simulink model "TRMS_Model"  (R2023b)
settings: Solver=FixedStepAuto  StartTime=0.0  StopTime=70  FixedStep=1e-5  RelTol=1e-3
libraries: slpidlib x2
settings Model: Creator=user  LastModifiedBy=user

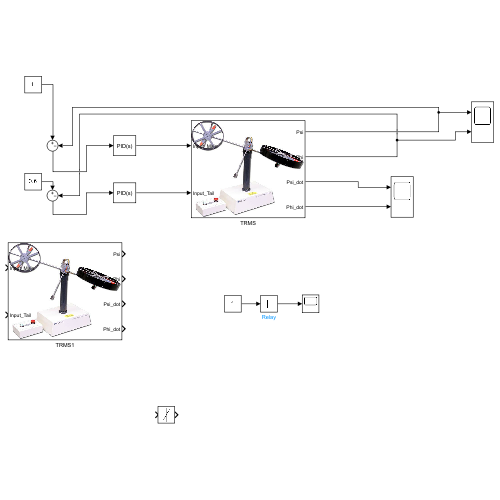
[thumbnail: Simulink's stored preview of the top-level diagram]
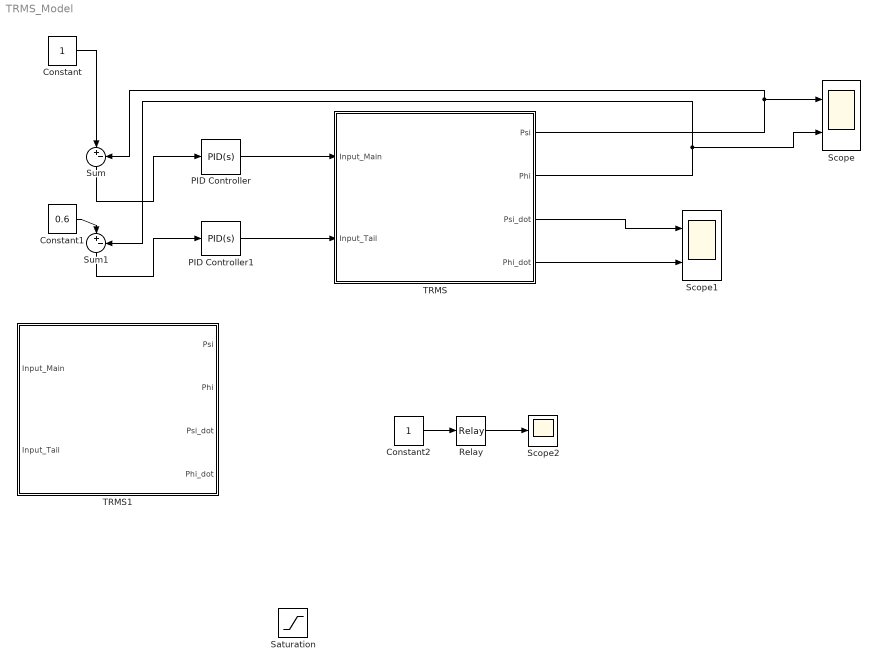
== system TRMS_Model ==
  Constant : Constant
  Constant1 : Constant  Value=0.6
  Constant2 : Constant
  PID Controller : slpidlib/PID Controller  Controller=PID  Form=Parallel  TimeDomain=Continuous-time  UseExternalTs=off  SampleTime=-1  IntegratorMethod=Forward Euler  FilterMethod=Forward Euler  ControllerParametersSource=internal  P=0  I=0.40844029645165  UseKiTs=off  D=0  N=100  UseFilter=on  TunerSelectOption=Transfer Function Based (PID Tuner App)  InitialConditionSource=internal  InitialConditionForIntegrator=0  InitialConditionForFilter=0  DifferentiatorICPrevScaledInput=0  ExternalReset=none  TrackingMode=off  Kt=1  LimitOutput=off  SatLimitsSource=internal  UpperSaturationLimit=inf  LowerSaturationLimit=-inf  LinearizeAsGain=on  AntiWindupMode=none  Kb=1  LimitIntegrator=off  UpperIntegratorSaturationLimit=inf  LowerIntegratorSaturationLimit=-inf  POutMin=[]  POutMax=[]  IOutMin=[]  IOutMax=[]  DOutMin=[]  DOutMax=[]  NOutMin=[]  NOutMax=[]  SumOutMin=[]  SumOutMax=[]  SaturationOutMin=[]  SaturationOutMax=[]  PParamMin=[]  PParamMax=[]  IParamMin=[]  IParamMax=[]  DParamMin=[]  DParamMax=[]  NParamMin=[]  NParamMax=[]  KbParamMin=[]  KbParamMax=[]  KtParamMin=[]  KtParamMax=[]  KbOutMin=[]  KbOutMax=[]  KtOutMin=[]  KtOutMax=[]  IntegratorOutMin=[]  IntegratorOutMax=[]  FilterOutMin=[]  FilterOutMax=[]  SumI1OutMin=[]  SumI1OutMax=[]  SumI2OutMin=[]  SumI2OutMax=[]  SumI3OutMin=[]  SumI3OutMax=[]  SumI4OutMin=[]  SumI4OutMax=[]  SumDOutMin=[]  SumDOutMax=[]  DifferentiatorOutMin=[]  DifferentiatorOutMax=[]  FilterDiffOutCoefMin=[]  FilterDiffOutCoefMax=[]  ReciprocalOutMin=[]  ReciprocalOutMax=[]  SumDenOutMin=[]  SumDenOutMax=[]  SumNumOutMin=[]  SumNumOutMax=[]  DivideOutMin=[]  DivideOutMax=[]  UdiffTsProdOutMin=[]  UdiffTsProdOutMax=[]  NTsProdOutMin=[]  NTsProdOutMax=[]  UintegralTsProdOutMin=[]  UintegralTsProdOutMax=[]  UngainTsProdOutMin=[]  UngainTsProdOutMax=[]  ClampingZeroOutDataTypeStr=Inherit: Inherit via back propagation  ClampingZeroOutMin=[]  ClampingZeroOutMax=[]  FilterDenConstantOutDataTypeStr=Inherit: Inherit via back propagation  FilterDenConstantOutMin=[]  FilterDenConstantOutMax=[]  PCopyOutDataTypeStr=Inherit: Inherit via back propagation  PCopyOutMin=[]  PCopyOutMax=[]  NCopyOutDataTypeStr=Inherit: Inherit via back propagation  NCopyOutMin=[]  NCopyOutMax=[]  IntegratorContinuousStateAttributes=''  IntegratorStateMustResolveToSignalObject=off  IntegratorRTWStateStorageClass=Auto  FilterContinuousStateAttributes=''  FilterStateMustResolveToSignalObject=off  FilterRTWStateStorageClass=Auto  ParallelPVariant=InternalParameters  IdealPVariant=Disabled  IVariant=InternalParameters  DVariant=InternalParameters  IntegratorVariant=Continuous  SatVariant=Disabled  AWVariant=Passthrough  PCopyVariant=Disabled  TRVariant=Disabled  FdbkBlocksVariant=Forward  IdealPFdbkVariant=Disabled  SatFdbkVariant=Disabled  DerivativeFilterVariant=ContFilter  NVariant=InternalParameters  NCopyVariant=Disabled  FilterICVariant=InternalICsFilter  IntegratorICVariant=InternalICs  ExternalResetVariant=Disabled  TRSumVariant=Passthrough  SumFdbkVariant=Disabled  SumVariant=Sum_PID  TsampFilterVariant=InternalTs  TsampNgainVariant=Passthrough  TsampIntegralVariant=Disabled_SignalSpec  ExternalSaturationOutDataTypeStr=Inherit: Same as second input
  PID Controller1 : slpidlib/PID Controller  Controller=PID  Form=Parallel  TimeDomain=Continuous-time  UseExternalTs=off  SampleTime=-1  IntegratorMethod=Forward Euler  FilterMethod=Forward Euler  ControllerParametersSource=internal  P=4.51040061904311  I=0.763929883616639  UseKiTs=off  D=4.55570625912268  N=321.160537839472  UseFilter=on  TunerSelectOption=Transfer Function Based (PID Tuner App)  InitialConditionSource=internal  InitialConditionForIntegrator=0  InitialConditionForFilter=0  DifferentiatorICPrevScaledInput=0  ExternalReset=none  TrackingMode=off  Kt=1  LimitOutput=off  SatLimitsSource=internal  UpperSaturationLimit=inf  LowerSaturationLimit=-inf  LinearizeAsGain=on  AntiWindupMode=none  Kb=1  LimitIntegrator=off  UpperIntegratorSaturationLimit=inf  LowerIntegratorSaturationLimit=-inf  POutMin=[]  POutMax=[]  IOutMin=[]  IOutMax=[]  DOutMin=[]  DOutMax=[]  NOutMin=[]  NOutMax=[]  SumOutMin=[]  SumOutMax=[]  SaturationOutMin=[]  SaturationOutMax=[]  PParamMin=[]  PParamMax=[]  IParamMin=[]  IParamMax=[]  DParamMin=[]  DParamMax=[]  NParamMin=[]  NParamMax=[]  KbParamMin=[]  KbParamMax=[]  KtParamMin=[]  KtParamMax=[]  KbOutMin=[]  KbOutMax=[]  KtOutMin=[]  KtOutMax=[]  IntegratorOutMin=[]  IntegratorOutMax=[]  FilterOutMin=[]  FilterOutMax=[]  SumI1OutMin=[]  SumI1OutMax=[]  SumI2OutMin=[]  SumI2OutMax=[]  SumI3OutMin=[]  SumI3OutMax=[]  SumI4OutMin=[]  SumI4OutMax=[]  SumDOutMin=[]  SumDOutMax=[]  DifferentiatorOutMin=[]  DifferentiatorOutMax=[]  FilterDiffOutCoefMin=[]  FilterDiffOutCoefMax=[]  ReciprocalOutMin=[]  ReciprocalOutMax=[]  SumDenOutMin=[]  SumDenOutMax=[]  SumNumOutMin=[]  SumNumOutMax=[]  DivideOutMin=[]  DivideOutMax=[]  UdiffTsProdOutMin=[]  UdiffTsProdOutMax=[]  NTsProdOutMin=[]  NTsProdOutMax=[]  UintegralTsProdOutMin=[]  UintegralTsProdOutMax=[]  UngainTsProdOutMin=[]  UngainTsProdOutMax=[]  ClampingZeroOutDataTypeStr=Inherit: Inherit via back propagation  ClampingZeroOutMin=[]  ClampingZeroOutMax=[]  FilterDenConstantOutDataTypeStr=Inherit: Inherit via back propagation  FilterDenConstantOutMin=[]  FilterDenConstantOutMax=[]  PCopyOutDataTypeStr=Inherit: Inherit via back propagation  PCopyOutMin=[]  PCopyOutMax=[]  NCopyOutDataTypeStr=Inherit: Inherit via back propagation  NCopyOutMin=[]  NCopyOutMax=[]  IntegratorContinuousStateAttributes=''  IntegratorStateMustResolveToSignalObject=off  IntegratorRTWStateStorageClass=Auto  FilterContinuousStateAttributes=''  FilterStateMustResolveToSignalObject=off  FilterRTWStateStorageClass=Auto  ParallelPVariant=InternalParameters  IdealPVariant=Disabled  IVariant=InternalParameters  DVariant=InternalParameters  IntegratorVariant=Continuous  SatVariant=Disabled  AWVariant=Passthrough  PCopyVariant=Disabled  TRVariant=Disabled  FdbkBlocksVariant=Forward  IdealPFdbkVariant=Disabled  SatFdbkVariant=Disabled  DerivativeFilterVariant=ContFilter  NVariant=InternalParameters  NCopyVariant=Disabled  FilterICVariant=InternalICsFilter  IntegratorICVariant=InternalICs  ExternalResetVariant=Disabled  TRSumVariant=Passthrough  SumFdbkVariant=Disabled  SumVariant=Sum_PID  TsampFilterVariant=InternalTs  TsampNgainVariant=Passthrough  TsampIntegralVariant=Disabled_SignalSpec  ExternalSaturationOutDataTypeStr=Inherit: Same as second input
  Relay : Relay  OnSwitchValue=0.01  OffSwitchValue=-0.01  OffOutputValue=-1
  Saturation : Saturate
  Scope : Scope  NumInputPorts=2
  Scope1 : Scope  NumInputPorts=2
  Scope2 : Scope
  Sum : Sum  Inputs=|+-
  Sum1 : Sum  Inputs=|+-
  TRMS : Subsystem
      mask Display: image('Twin-Rotor-MIMO-System.png');
  TRMS1 : Subsystem
      mask Display: image('Twin-Rotor-MIMO-System.png');
  wires:
  PID Controller/1 -> TRMS/1(Input_Main)
  Sum/1 -> PID Controller/1
  Constant/1 -> Sum/1
  TRMS/1(Psi) -> Scope/1, Sum/2
  PID Controller1/1 -> TRMS/2(Input_Tail)
  Constant1/1 -> Sum1/1
  Sum1/1 -> PID Controller1/1
  TRMS/2(Phi) -> Scope/2, Sum1/2
  TRMS/3(Psi_dot) -> Scope1/1
  TRMS/4(Phi_dot) -> Scope1/2
  Relay/1 -> Scope2/1
  Constant2/1 -> Relay/1

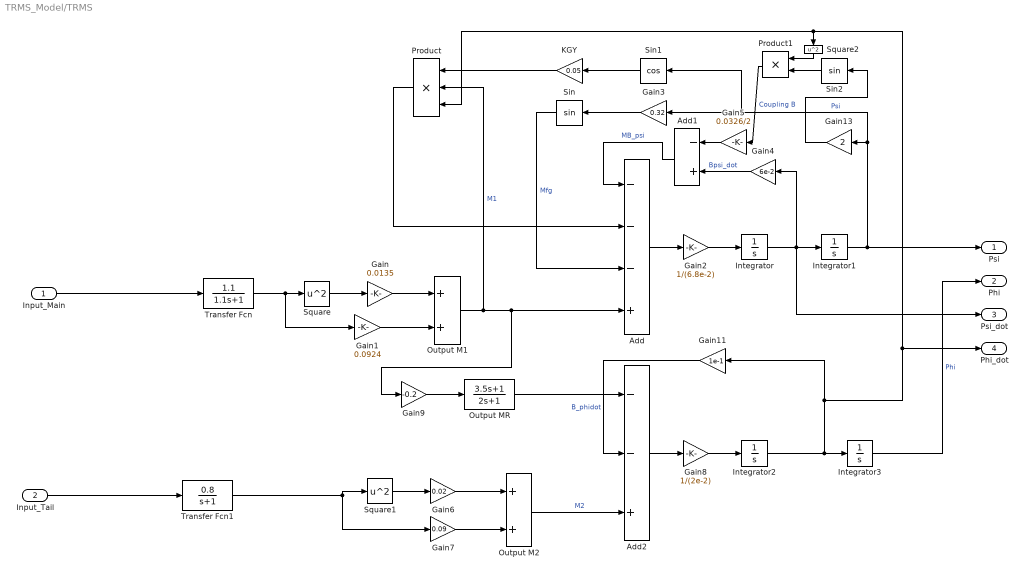
== system TRMS_Model/TRMS ==
  Input_Main : Inport
  Input_Tail : Inport  Port=2
  Add : Sum  Inputs=---+
  Add1 : Sum  Inputs=-+
  Add2 : Sum  Inputs=--+
  Gain : Gain  Gain=0.0135
  Gain1 : Gain  Gain=0.0924
  Gain11 : Gain  Gain=1e-1
  Gain13 : Gain  Gain=2
  Gain2 : Gain  Gain=1/(6.8e-2)
  Gain3 : Gain  Gain=0.32
  Gain4 : Gain  Gain=6e-2
  Gain5 : Gain  Gain=0.0326/2
  Gain6 : Gain  Gain=0.02
  Gain7 : Gain  Gain=0.09
  Gain8 : Gain  Gain=1/(2e-2)
  Gain9 : Gain  Gain=-0.2
  Integrator{,1..3} (4 alike) : Integrator
  KGY : Gain  Gain=0.05
  Output M1 : Sum
  Output M2 : Sum
  Output MR : TransferFcn  Numerator=[3.5 1]  Denominator=[2 1]
  Product : Product  Inputs=3
  Product1 : Product
  Sin : Trigonometry
  Sin1 : Trigonometry  Operator=cos
  Sin2 : Trigonometry
  Square : Math  Operator=square
  Square1 : Math  Operator=square
  Square2 : Math  Operator=square
  Transfer Fcn : TransferFcn  Numerator=[1.1]  Denominator=[1.1 1]
  Transfer Fcn1 : TransferFcn  Numerator=[0.8]  Denominator=[1 1]
  Psi : Outport
  Phi : Outport  Port=2
  Psi_dot : Outport  Port=3
  Phi_dot : Outport  Port=4
  wires:
  Integrator2/1 -> Phi_dot/1, Product/3, Square2/1, Gain11/1, Integrator3/1
  Product1/1 -> Gain5/1  "Coupling B"
  Add1/1 -> Add/1  "MB_psi"
  Integrator1/1 -> Psi/1, Gain13/1, Sin1/1, Gain3/1  "Psi"
  Sin2/1 -> Product1/2
  Product/1 -> Add/2
  Transfer Fcn/1 -> Square/1, Gain1/1
  Square1/1 -> Gain6/1
  Gain3/1 -> Sin/1
  Add/1 -> Gain2/1
  Gain1/1 -> Output M1/2
  Square/1 -> Gain/1
  Gain13/1 -> Sin2/1
  Transfer Fcn1/1 -> Gain7/1, Square1/1
  Integrator/1 -> Psi_dot/1, Gain4/1, Integrator1/1
  Gain/1 -> Output M1/1
  Gain9/1 -> Output MR/1
  Gain6/1 -> Output M2/1
  Output M2/1 -> Add2/3  "M2"
  Output M1/1 -> Gain9/1, Add/4, Product/2  "M1"
  Add2/1 -> Gain8/1
  Sin1/1 -> KGY/1
  Gain2/1 -> Integrator/1
  KGY/1 -> Product/1
  Gain11/1 -> Add2/2  "B_phidot"
  Gain7/1 -> Output M2/2
  Output MR/1 -> Add2/1
  Gain8/1 -> Integrator2/1
  Gain4/1 -> Add1/2  "Bpsi_dot"
  Gain5/1 -> Add1/1
  Input_Main/1 -> Transfer Fcn/1
  Sin/1 -> Add/3  "Mfg"
  Square2/1 -> Product1/1
  Input_Tail/1 -> Transfer Fcn1/1
  Integrator3/1 -> Phi/1  "Phi"

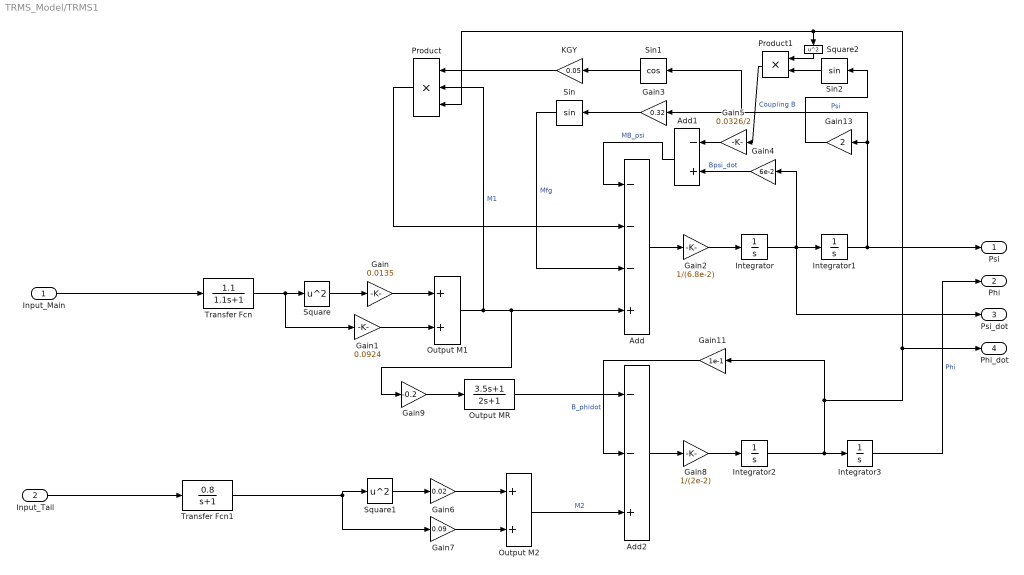
== system TRMS_Model/TRMS1 ==
  Input_Main : Inport
  Input_Tail : Inport  Port=2
  Add : Sum  Inputs=---+
  Add1 : Sum  Inputs=-+
  Add2 : Sum  Inputs=--+
  Gain : Gain  Gain=0.0135
  Gain1 : Gain  Gain=0.0924
  Gain11 : Gain  Gain=1e-1
  Gain13 : Gain  Gain=2
  Gain2 : Gain  Gain=1/(6.8e-2)
  Gain3 : Gain  Gain=0.32
  Gain4 : Gain  Gain=6e-2
  Gain5 : Gain  Gain=0.0326/2
  Gain6 : Gain  Gain=0.02
  Gain7 : Gain  Gain=0.09
  Gain8 : Gain  Gain=1/(2e-2)
  Gain9 : Gain  Gain=-0.2
  Integrator{,1..3} (4 alike) : Integrator
  KGY : Gain  Gain=0.05
  Output M1 : Sum
  Output M2 : Sum
  Output MR : TransferFcn  Numerator=[3.5 1]  Denominator=[2 1]
  Product : Product  Inputs=3
  Product1 : Product
  Sin : Trigonometry
  Sin1 : Trigonometry  Operator=cos
  Sin2 : Trigonometry
  Square : Math  Operator=square
  Square1 : Math  Operator=square
  Square2 : Math  Operator=square
  Transfer Fcn : TransferFcn  Numerator=[1.1]  Denominator=[1.1 1]
  Transfer Fcn1 : TransferFcn  Numerator=[0.8]  Denominator=[1 1]
  Psi : Outport
  Phi : Outport  Port=2
  Psi_dot : Outport  Port=3
  Phi_dot : Outport  Port=4
  wires:
  Integrator3/1 -> Phi/1  "Phi"
  Input_Tail/1 -> Transfer Fcn1/1
  Square2/1 -> Product1/1
  Sin/1 -> Add/3  "Mfg"
  Input_Main/1 -> Transfer Fcn/1
  Gain5/1 -> Add1/1
  Gain4/1 -> Add1/2  "Bpsi_dot"
  Gain8/1 -> Integrator2/1
  Output MR/1 -> Add2/1
  Gain7/1 -> Output M2/2
  Gain11/1 -> Add2/2  "B_phidot"
  KGY/1 -> Product/1
  Gain2/1 -> Integrator/1
  Sin1/1 -> KGY/1
  Add2/1 -> Gain8/1
  Output M1/1 -> Product/2, Add/4, Gain9/1  "M1"
  Output M2/1 -> Add2/3  "M2"
  Gain6/1 -> Output M2/1
  Gain9/1 -> Output MR/1
  Gain/1 -> Output M1/1
  Integrator/1 -> Integrator1/1, Gain4/1, Psi_dot/1
  Transfer Fcn1/1 -> Square1/1, Gain7/1
  Gain13/1 -> Sin2/1
  Square/1 -> Gain/1
  Gain1/1 -> Output M1/2
  Add/1 -> Gain2/1
  Gain3/1 -> Sin/1
  Square1/1 -> Gain6/1
  Transfer Fcn/1 -> Gain1/1, Square/1
  Product/1 -> Add/2
  Sin2/1 -> Product1/2
  Integrator1/1 -> Gain3/1, Sin1/1, Gain13/1, Psi/1  "Psi"
  Add1/1 -> Add/1  "MB_psi"
  Product1/1 -> Gain5/1  "Coupling B"
  Integrator2/1 -> Integrator3/1, Gain11/1, Square2/1, Product/3, Phi_dot/1
